simulink model "PhasePlaneControl"  (R2021a)
settings: configuration reference "RPi_ControlRate" (kept outside this file)
settings Model: Creator=Andy  LastModifiedBy=Andy
settings ConfigSetRef: SourceName=RPi_ControlRate  SourceLocation=Base Workspace

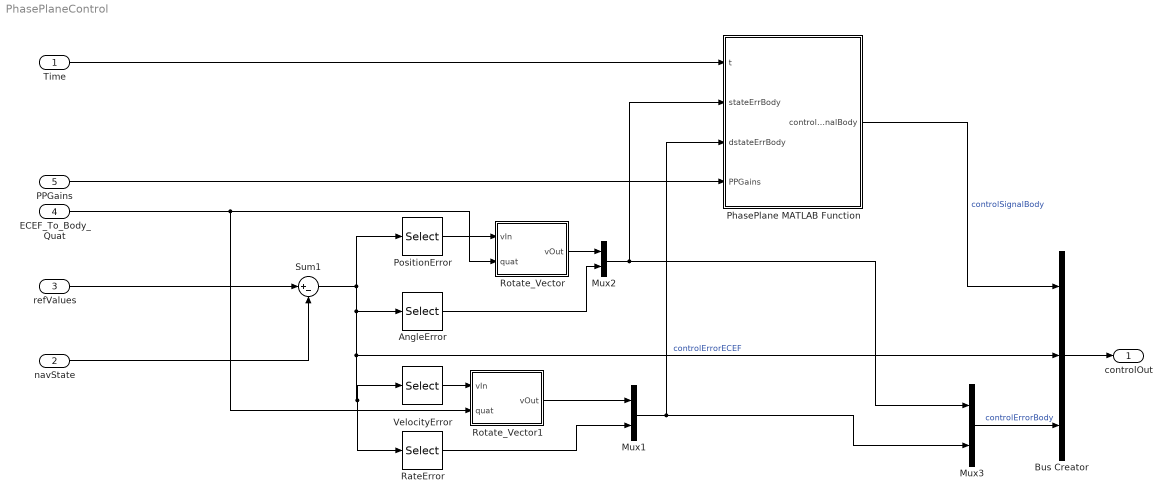
== system PhasePlaneControl ==
  Time : Inport
  navState : Inport  Port=2  PortDimensions=12
  refValues : Inport  Port=3  PortDimensions=12
  ECEF_To_Body_Quat : Inport  Port=4  OutDataTypeStr=double  PortDimensions=4
  PPGains : Inport  Port=5  PortDimensions=12
  AngleError : Selector  IndexOptions=Index vector (dialog)  Indices=[4:6]  OutputSizes=1
  Bus Creator : BusCreator  Inputs=3  OutDataTypeStr=Bus: ControlOutBus
      settings: InheritFromInputs=off
  Mux1 : Mux  Inputs=2
  Mux2 : Mux  Inputs=2
  Mux3 : Mux  Inputs=2
  PhasePlane MATLAB Function : MATLAB Function  TreatAsAtomicUnit=on
  PositionError : Selector  IndexOptions=Index vector (dialog)  Indices=[1:3]  OutputSizes=1
  RateError : Selector  IndexOptions=Index vector (dialog)  Indices=[10:12]  OutputSizes=1
  Rotate_Vector : MATLAB Function  TreatAsAtomicUnit=on
  Rotate_Vector1 : MATLAB Function  TreatAsAtomicUnit=on
  Sum1 : Sum  Inputs=|+-
  VelocityError : Selector  IndexOptions=Index vector (dialog)  Indices=[7:9]  OutputSizes=1
  controlOut : Outport  OutDataTypeStr=Bus: ControlOutBus  VectorParamsAs1DForOutWhenUnconnected=off
  wires:
  PhasePlane MATLAB Function/1(controlSignalBody) -> Bus Creator/1  "controlSignalBody"
  Bus Creator/1 -> controlOut/1
  Rotate_Vector/1(vOut) -> Mux2/1
  navState/1 -> Sum1/2
  PositionError/1 -> Rotate_Vector/1(vIn)
  Mux2/1 -> PhasePlane MATLAB Function/2(stateErrBody), Mux3/1
  VelocityError/1 -> Rotate_Vector1/1(vIn)
  AngleError/1 -> Mux2/2
  refValues/1 -> Sum1/1
  Mux1/1 -> PhasePlane MATLAB Function/3(dstateErrBody), Mux3/2
  Sum1/1 -> RateError/1, VelocityError/1, Bus Creator/2, AngleError/1, PositionError/1  "controlErrorECEF"
  ECEF_To_Body_Quat/1 -> Rotate_Vector/2(quat), Rotate_Vector1/2(quat)
  RateError/1 -> Mux1/2
  Rotate_Vector1/1(vOut) -> Mux1/1
  Mux3/1 -> Bus Creator/3  "controlErrorBody"
  PPGains/1 -> PhasePlane MATLAB Function/4(PPGains)
  Time/1 -> PhasePlane MATLAB Function/1(t)

== matlab function PhasePlaneControl/Rotate_Vector ==
  data: vIn input; vOut output; quat input
function vOut  = fcn(vIn,quat)


vOut = quatrotate(vIn,quat')';

== matlab function PhasePlaneControl/PhasePlane MATLAB Function ==
  data: t input; controlSignalBody output; stateErrBody input; dstateErrBody input; PPGains input
function controlSignalBody  = callPhasePlaneControl(t,stateErrBody,dstateErrBody,PPGains)



controlSignalBody = zeros(6,1);

% X Translation
drift_channel_db    = PPGains(1);
drift_channel_rate  = PPGains(2);
drift_channel_width = PPGains(3);  
max_cmd             = PPGains(4);
controlSignalBody(1) = phasePlaneControl(stateErrBody(1),dstateErrBody(1),...
                                   drift_channel_db,drift_channel_rate, ...
                                   drift_channel_width, max_cmd);
% Y Translation
drift_channel_db    = PPGains(5);
drift_channel_rate  = PPGains(6);
drift_channel_width = PPGains(7);  
max_cmd             = PPGains(8);
controlSignalBody(2) = phasePlaneControl(stateErrBody(2),dstateErrBody(2),...
                                   drift_channel_db,drift_channel_rate, ...
                                   drift_channel_width, max_cmd);

% Z Rotation
drift_channel_db    = PPGains(9);
drift_channel_rate  = PPGains(10);
drift_channel_width = PPGains(11);  
max_cmd             = PPGains(12);
controlSignalBody(6) = phasePlaneControl(stateErrBody(6),dstateErrBody(6),...
                                   drift_channel_db,drift_channel_rate, ...
                                   drift_channel_width, max_cmd);
                               
controlSignalBody = -1*controlSignalBody;

== matlab function PhasePlaneControl/Rotate_Vector1 ==
  data: vIn input; vOut output; quat input
function vOut  = fcn(vIn,quat)


vOut = quatrotate(vIn,quat')';
